simulink model "btp_gas_networkmodel"  (R2020a)
settings: Solver=VariableStepAuto  StartTime=0.0  StopTime=1e5  RelTol=1e-3
PreLoadFcn:
  | building_length = 15; % m
  | building_width = 10; % m
  | building_height = 2.5; % m
  | 
  | wall_thickness = 0.2; % m
  | wall_density = 2000; % kg/m^3
  | wall_specific_heat = 840; % J/(kg*K)
  | wall_conductivity = 0.04; % W/(m*K)
  | wall_heat_transfer_coeff_internal = 25; % W/(m^2*K)
  | wall_heat_transfer_coeff_external = 35; % W/(m^2*K)
  | 
  | roof_thickness = 0.2; % m
  | roof_density = 2000; % kg/m^3
  | roof_specific_heat = 840; % J/(kg*K)
  | roof_conductivity = 0.035; % W/(m*K)
  | roof_heat_transfer_coeff_internal = 10; % W/(m^2*K)
  | roof_heat_transfer_coeff_external = 30; % W/(m^2*K)
  | 
  | floor_thickness = 0.1; % m
  | floor_conductivity = 0.15; % W/(m*K)
  | floor_heat_transfer_coeff_internal = 15; % W/(m^2*K)
  | 
  | door_area = 2*0.6; % m^2
  | 
  | duct_area = 0.1^2; % m^2
  | 
  | fan_setting_table = 0 : 4; % 1
  | fan_flow_rate_table = [0 0.08 0.12 0.16 0.2]; % kg/s
  | 
  | initial_temperature = 35; % degC
  | ground_temperature = 25; % degC
  | 
  | flow_reversal_Mach = 1e-5; % 1
InitFcn:
  | zone_volume = building_length * building_width * building_height / 4; % m^3
  | zone_flow_area = 0.7 * building_height * (building_length + building_width) / 4; % m^2
undefined symbols (not defined in the file): sigbuilder_block
libraries: fl_lib x49, nesl_utility x15
(part 2 of 2)

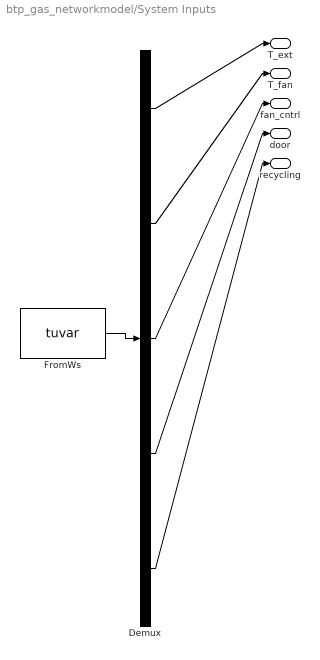
== system btp_gas_networkmodel/System Inputs ==
  Demux : Demux  Tag=STV Demux  Outputs=5
      settings: DisplayOption=none
  FromWs : FromWorkspace  Tag=STV FromWs  VariableName=tuvar
      SigBuilderData=|
      | common.afterFinalStr = 'Extrapolate'
      | common.sampleTime = 0
      | dataSet(1).timeRange = [0 100000]
      | dataSet(1).name = 'Fan Control'
      | dataSet(2).timeRange = [0 100000]
      | dataSet(2).name = 'Fan Temperature'
      | dataSet(3).timeRange = [0 100000]
      | dataSet(3).name = 'Disturbances'
      | sbobj.Groups(1).Name = 'Fan Control'
      | sbobj.Groups(1).Signals(1).Name = 'T_ext'
      | sbobj.Groups(1).Signals(1).XData = [0 100000]
      | sbobj.Groups(1).Signals(1).YData = [35 35]
      | sbobj.Groups(1).Signals(2).Name = 'T_fan'
      | sbobj.Groups(1).Signals(2).XData = [0 100000]
      | sbobj.Groups(1).Signals(2).YData = [20 20]
      | sbobj.Groups(1).Signals(3).Name = 'fan_cntrl'
      | sbobj.Groups(1).Signals(3).XData = [0 20000 20000 40000 40000 60000 80000 100000]
      | sbobj.Groups(1).Signals(3).YData = [1 1 2 2 1 1 1 1]
      | sbobj.Groups(1).Signals(4).Name = 'door'
      | sbobj.Groups(1).Signals(4).XData = [0 100000]
      | sbobj.Groups(1).Signals(4).YData = [0 0]
      | sbobj.Groups(1).Signals(5).Name = 'recycling'
      | sbobj.Groups(1).Signals(5).XData = [0 100000]
      | sbobj.Groups(1).Signals(5).YData = [0 0]
      | sbobj.Groups(1).TimeRange = [0 100000]
      | sbobj.Groups(2).Name = 'Fan Temperature'
      | sbobj.Groups(2).Signals(1).Name = 'T_ext'
      | sbobj.Groups(2).Signals(1).XData = [0 100000]
      | sbobj.Groups(2).Signals(1).YData = [35 35]
      | sbobj.Groups(2).Signals(2).Name = 'T_fan'
      | sbobj.Groups(2).Signals(2).XData = [0 20000 20000 40000 40000 60000 60000 80000 80000 100000]
      | sbobj.Groups(2).Signals(2).YData = [20 20 15 15 20 20 35 35 20 20]
      | sbobj.Groups(2).Signals(3).Name = 'fan_cntrl'
      | sbobj.Groups(2).Signals(3).XData = [0 100000]
      | sbobj.Groups(2).Signals(3).YData = [1 1]
      | sbobj.Groups(2).Signals(4).Name = 'door'
      | sbobj.Groups(2).Signals(4).XData = [0 100000]
      | sbobj.Groups(2).Signals(4).YData = [0 0]
      | sbobj.Groups(2).Signals(5).Name = 'recycling'
      | sbobj.Groups(2).Signals(5).XData = [0 100000]
      | sbobj.Groups(2).Signals(5).YData = [0 0]
      | sbobj.Groups(2).TimeRange = [0 100000]
      | sbobj.Groups(3).Name = 'Disturbances'
      | sbobj.Groups(3).Signals(1).Name = 'T_ext'
      | sbobj.Groups(3).Signals(1).XData = [0 100000]
      | sbobj.Groups(3).Signals(1).YData = [35 35]
      | sbobj.Groups(3).Signals(2).Name = 'T_fan'
      | sbobj.Groups(3).Signals(2).XData = [0 100000]
      | sbobj.Groups(3).Signals(2).YData = [20 20]
      | sbobj.Groups(3).Signals(3).Name = 'fan_cntrl'
      | sbobj.Groups(3).Signals(3).XData = [0 100000]
      | sbobj.Groups(3).Signals(3).YData = [1 1]
      | sbobj.Groups(3).Signals(4).Name = 'door'
      | sbobj.Groups(3).Signals(4).XData = [0 20000 30000 40000 100000]
      | sbobj.Groups(3).Signals(4).YData = [0 0 1 0 0]
      | sbobj.Groups(3).Signals(5).Name = 'recycling'
      | sbobj.Groups(3).Signals(5).XData = [0 60000 60000 80000 80000 100000]
      | sbobj.Groups(3).Signals(5).YData = [0 0 0.5 0.5 0 0]
      | sbobj.Groups(3).TimeRange = [0 100000]
  T_ext : Outport  Tag=STV Outport  VectorParamsAs1DForOutWhenUnconnected=off
  T_fan : Outport  Tag=STV Outport  Port=2  VectorParamsAs1DForOutWhenUnconnected=off
  fan_cntrl : Outport  Tag=STV Outport  Port=3  VectorParamsAs1DForOutWhenUnconnected=off
  door : Outport  Tag=STV Outport  Port=4  VectorParamsAs1DForOutWhenUnconnected=off
  recycling : Outport  Tag=STV Outport  Port=5  VectorParamsAs1DForOutWhenUnconnected=off
  wires:
  FromWs/1 -> Demux/1
  Demux/1 -> T_ext/1
  Demux/2 -> T_fan/1
  Demux/3 -> fan_cntrl/1
  Demux/4 -> door/1
  Demux/5 -> recycling/1

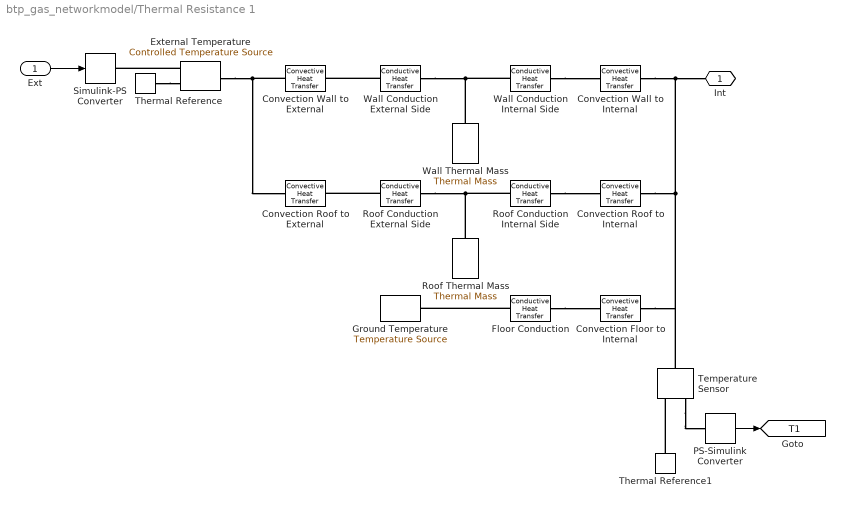
== system btp_gas_networkmodel/Thermal Resistance 1 ==
  Ext : Inport
  Convection Floor to Internal : fl_lib/Thermal/Thermal Elements/Convective Heat Transfer  area=floor_area m^2  heat_tr_coeff=floor_heat_transfer_coeff_internal W/(m^2 * K)  T_specify=off  T_priority=None  T=0 K  T_nominal_specify=off  T_nominal_unit=K  T_nominal_value=1  Q_specify=off  Q_priority=None  Q=0 W  Q_nominal_specify=off  Q_nominal_unit=W  Q_nominal_value=1
  Convection Roof to External : fl_lib/Thermal/Thermal Elements/Convective Heat Transfer  area=roof_area m^2  heat_tr_coeff=roof_heat_transfer_coeff_external W/(m^2 * K)  T_specify=off  T_priority=None  T=0 K  T_nominal_specify=off  T_nominal_unit=K  T_nominal_value=1  Q_specify=off  Q_priority=None  Q=0 W  Q_nominal_specify=off  Q_nominal_unit=W  Q_nominal_value=1
  Convection Roof to Internal : fl_lib/Thermal/Thermal Elements/Convective Heat Transfer  area=roof_area m^2  heat_tr_coeff=roof_heat_transfer_coeff_internal W/(m^2 * K)  T_specify=off  T_priority=None  T=0 K  T_nominal_specify=off  T_nominal_unit=K  T_nominal_value=1  Q_specify=off  Q_priority=None  Q=0 W  Q_nominal_specify=off  Q_nominal_unit=W  Q_nominal_value=1
  Convection Wall to External : fl_lib/Thermal/Thermal Elements/Convective Heat Transfer  area=wall_area m^2  heat_tr_coeff=wall_heat_transfer_coeff_external W/(m^2 * K)  T_specify=off  T_priority=None  T=0 K  T_nominal_specify=off  T_nominal_unit=K  T_nominal_value=1  Q_specify=off  Q_priority=None  Q=0 W  Q_nominal_specify=off  Q_nominal_unit=W  Q_nominal_value=1
  Convection Wall to Internal : fl_lib/Thermal/Thermal Elements/Convective Heat Transfer  area=wall_area m^2  heat_tr_coeff=wall_heat_transfer_coeff_internal W/(m^2 * K)  T_specify=off  T_priority=None  T=0 K  T_nominal_specify=off  T_nominal_unit=K  T_nominal_value=1  Q_specify=off  Q_priority=None  Q=0 W  Q_nominal_specify=off  Q_nominal_unit=W  Q_nominal_value=1
  External Temperature : fl_lib/Thermal/Thermal Sources/Controlled Temperature Source
  Floor Conduction : fl_lib/Thermal/Thermal Elements/Conductive Heat Transfer  area=floor_area m^2  thickness=floor_thickness m  th_cond=floor_conductivity W/(m*K)  T_specify=off  T_priority=None  T=0 K  T_nominal_specify=off  T_nominal_unit=K  T_nominal_value=1  Q_specify=off  Q_priority=None  Q=0 W  Q_nominal_specify=off  Q_nominal_unit=W  Q_nominal_value=1
  Ground Temperature : fl_lib/Thermal/Thermal Sources/Temperature Source  temperature=ground_temperature degC
  PS-Simulink Converter : nesl_utility/PS-Simulink Converter  PhysicalDomain=network_engine_domain  SubClassName=ps_output  LeftPortType=input  RightPortType=output  PseudoPeriodic=off  Frequencies=[]  Unit=degC  AffineConversion=on
  Roof Conduction External Side : fl_lib/Thermal/Thermal Elements/Conductive Heat Transfer  area=roof_area m^2  thickness=roof_thickness / 2 m  th_cond=roof_conductivity W/(m*K)  T_specify=off  T_priority=None  T=0 K  T_nominal_specify=off  T_nominal_unit=K  T_nominal_value=1  Q_specify=off  Q_priority=None  Q=0 W  Q_nominal_specify=off  Q_nominal_unit=W  Q_nominal_value=1
  Roof Conduction Internal Side : fl_lib/Thermal/Thermal Elements/Conductive Heat Transfer  area=roof_area m^2  thickness=roof_thickness / 2 m  th_cond=roof_conductivity W/(m*K)  T_specify=off  T_priority=None  T=0 K  T_nominal_specify=off  T_nominal_unit=K  T_nominal_value=1  Q_specify=off  Q_priority=None  Q=0 W  Q_nominal_specify=off  Q_nominal_unit=W  Q_nominal_value=1
  Roof Thermal Mass : fl_lib/Thermal/Thermal Elements/Thermal Mass  mass=roof_area * roof_thickness * wall_density kg  sp_heat=roof_specific_heat J/kg/K  T_specify=on  T_priority=High  T=roof_initial_temperature degC  T_nominal_specify=off  T_nominal_unit=K  T_nominal_value=1  Q_specify=off  Q_priority=None  Q=0 W  Q_nominal_specify=off  Q_nominal_unit=W  Q_nominal_value=1
  Simulink-PS Converter : nesl_utility/Simulink-PS Converter  PhysicalDomain=network_engine_domain  SubClassName=ps_input  LeftPortType=input  RightPortType=output  PseudoPeriodic=off  Frequencies=[]  NoiseDistribution=none  NoiseParameters=[]  Unit=degC  AffineConversion=on  FilteringAndDerivatives=provide  SimscapeFilterOrder=1  InputFilterTimeConstant=0.001  UdotUserProvided=0
  Temperature Sensor : fl_lib/Thermal/Thermal Sensors/Temperature Sensor
  Thermal Reference : fl_lib/Thermal/Thermal Elements/Thermal Reference
  Thermal Reference1 : fl_lib/Thermal/Thermal Elements/Thermal Reference
  Wall Conduction External Side : fl_lib/Thermal/Thermal Elements/Conductive Heat Transfer  area=wall_area m^2  thickness=wall_thickness / 2 m  th_cond=wall_conductivity W/(m*K)  T_specify=off  T_priority=None  T=0 K  T_nominal_specify=off  T_nominal_unit=K  T_nominal_value=1  Q_specify=off  Q_priority=None  Q=0 W  Q_nominal_specify=off  Q_nominal_unit=W  Q_nominal_value=1
  Wall Conduction Internal Side : fl_lib/Thermal/Thermal Elements/Conductive Heat Transfer  area=wall_area m^2  thickness=wall_thickness / 2 m  th_cond=wall_conductivity W/(m*K)  T_specify=off  T_priority=None  T=0 K  T_nominal_specify=off  T_nominal_unit=K  T_nominal_value=1  Q_specify=off  Q_priority=None  Q=0 W  Q_nominal_specify=off  Q_nominal_unit=W  Q_nominal_value=1
  Wall Thermal Mass : fl_lib/Thermal/Thermal Elements/Thermal Mass  mass=wall_area * wall_thickness * wall_density kg  sp_heat=wall_specific_heat J/kg/K  T_specify=on  T_priority=High  T=wall_initial_temperature degC  T_nominal_specify=off  T_nominal_unit=K  T_nominal_value=1  Q_specify=off  Q_priority=None  Q=0 W  Q_nominal_specify=off  Q_nominal_unit=W  Q_nominal_value=1
  Int : PMIOPort  Side=Right
  tag scope: T1=global
  wires:
  Ext/1 -> Simulink-PS Converter/1
  PS-Simulink Converter/1 -> [T1]
  connections:
  External Temperature/RConn1 -- Simulink-PS Converter/RConn1
  Wall Conduction Internal Side/RConn1 -- Convection Wall to Internal/LConn1
  Convection Roof to Internal/RConn1 -- Convection Floor to Internal/RConn1 -- Temperature Sensor/LConn1 -- Convection Wall to Internal/RConn1 -- Int/RConn1
  External Temperature/LConn1 -- Convection Wall to External/LConn1 -- Convection Roof to External/LConn1
  Wall Conduction External Side/LConn1 -- Convection Wall to External/RConn1
  Wall Thermal Mass/LConn1 -- Wall Conduction Internal Side/LConn1 -- Wall Conduction External Side/RConn1
  Roof Thermal Mass/LConn1 -- Roof Conduction Internal Side/LConn1 -- Roof Conduction External Side/RConn1
  Roof Conduction External Side/LConn1 -- Convection Roof to External/RConn1
  Roof Conduction Internal Side/RConn1 -- Convection Roof to Internal/LConn1
  Floor Conduction/RConn1 -- Convection Floor to Internal/LConn1
  Floor Conduction/LConn1 -- Ground Temperature/LConn1
  Thermal Reference1/LConn1 -- Temperature Sensor/RConn1
  Temperature Sensor/RConn2 -- PS-Simulink Converter/LConn1
  Thermal Reference/LConn1 -- External Temperature/RConn2

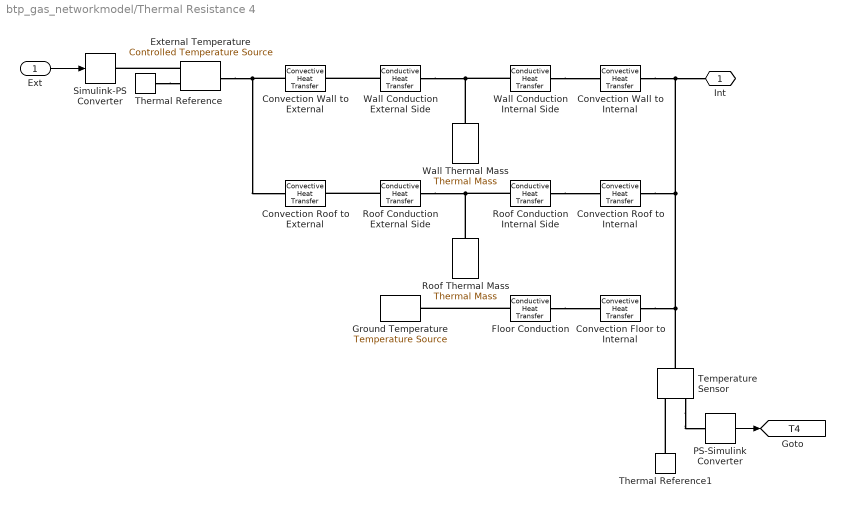
== system btp_gas_networkmodel/Thermal Resistance 4 ==
  Ext : Inport
  Convection Floor to Internal : fl_lib/Thermal/Thermal Elements/Convective Heat Transfer  area=floor_area m^2  heat_tr_coeff=floor_heat_transfer_coeff_internal W/(m^2 * K)  T_specify=off  T_priority=None  T=0 K  T_nominal_specify=off  T_nominal_unit=K  T_nominal_value=1  Q_specify=off  Q_priority=None  Q=0 W  Q_nominal_specify=off  Q_nominal_unit=W  Q_nominal_value=1
  Convection Roof to External : fl_lib/Thermal/Thermal Elements/Convective Heat Transfer  area=roof_area m^2  heat_tr_coeff=roof_heat_transfer_coeff_external W/(m^2 * K)  T_specify=off  T_priority=None  T=0 K  T_nominal_specify=off  T_nominal_unit=K  T_nominal_value=1  Q_specify=off  Q_priority=None  Q=0 W  Q_nominal_specify=off  Q_nominal_unit=W  Q_nominal_value=1
  Convection Roof to Internal : fl_lib/Thermal/Thermal Elements/Convective Heat Transfer  area=roof_area m^2  heat_tr_coeff=roof_heat_transfer_coeff_internal W/(m^2 * K)  T_specify=off  T_priority=None  T=0 K  T_nominal_specify=off  T_nominal_unit=K  T_nominal_value=1  Q_specify=off  Q_priority=None  Q=0 W  Q_nominal_specify=off  Q_nominal_unit=W  Q_nominal_value=1
  Convection Wall to External : fl_lib/Thermal/Thermal Elements/Convective Heat Transfer  area=wall_area m^2  heat_tr_coeff=wall_heat_transfer_coeff_external W/(m^2 * K)  T_specify=off  T_priority=None  T=0 K  T_nominal_specify=off  T_nominal_unit=K  T_nominal_value=1  Q_specify=off  Q_priority=None  Q=0 W  Q_nominal_specify=off  Q_nominal_unit=W  Q_nominal_value=1
  Convection Wall to Internal : fl_lib/Thermal/Thermal Elements/Convective Heat Transfer  area=wall_area m^2  heat_tr_coeff=wall_heat_transfer_coeff_internal W/(m^2 * K)  T_specify=off  T_priority=None  T=0 K  T_nominal_specify=off  T_nominal_unit=K  T_nominal_value=1  Q_specify=off  Q_priority=None  Q=0 W  Q_nominal_specify=off  Q_nominal_unit=W  Q_nominal_value=1
  External Temperature : fl_lib/Thermal/Thermal Sources/Controlled Temperature Source
  Floor Conduction : fl_lib/Thermal/Thermal Elements/Conductive Heat Transfer  area=floor_area m^2  thickness=floor_thickness m  th_cond=floor_conductivity W/(m*K)  T_specify=off  T_priority=None  T=0 K  T_nominal_specify=off  T_nominal_unit=K  T_nominal_value=1  Q_specify=off  Q_priority=None  Q=0 W  Q_nominal_specify=off  Q_nominal_unit=W  Q_nominal_value=1
  Ground Temperature : fl_lib/Thermal/Thermal Sources/Temperature Source  temperature=ground_temperature degC
  PS-Simulink Converter : nesl_utility/PS-Simulink Converter  PhysicalDomain=network_engine_domain  SubClassName=ps_output  LeftPortType=input  RightPortType=output  PseudoPeriodic=off  Frequencies=[]  Unit=degC  AffineConversion=on
  Roof Conduction External Side : fl_lib/Thermal/Thermal Elements/Conductive Heat Transfer  area=roof_area m^2  thickness=roof_thickness / 2 m  th_cond=roof_conductivity W/(m*K)  T_specify=off  T_priority=None  T=0 K  T_nominal_specify=off  T_nominal_unit=K  T_nominal_value=1  Q_specify=off  Q_priority=None  Q=0 W  Q_nominal_specify=off  Q_nominal_unit=W  Q_nominal_value=1
  Roof Conduction Internal Side : fl_lib/Thermal/Thermal Elements/Conductive Heat Transfer  area=roof_area m^2  thickness=roof_thickness / 2 m  th_cond=roof_conductivity W/(m*K)  T_specify=off  T_priority=None  T=0 K  T_nominal_specify=off  T_nominal_unit=K  T_nominal_value=1  Q_specify=off  Q_priority=None  Q=0 W  Q_nominal_specify=off  Q_nominal_unit=W  Q_nominal_value=1
  Roof Thermal Mass : fl_lib/Thermal/Thermal Elements/Thermal Mass  mass=roof_area * roof_thickness * wall_density kg  sp_heat=roof_specific_heat J/kg/K  T_specify=on  T_priority=High  T=roof_initial_temperature degC  T_nominal_specify=off  T_nominal_unit=K  T_nominal_value=1  Q_specify=off  Q_priority=None  Q=0 W  Q_nominal_specify=off  Q_nominal_unit=W  Q_nominal_value=1
  Simulink-PS Converter : nesl_utility/Simulink-PS Converter  PhysicalDomain=network_engine_domain  SubClassName=ps_input  LeftPortType=input  RightPortType=output  PseudoPeriodic=off  Frequencies=[]  NoiseDistribution=none  NoiseParameters=[]  Unit=degC  AffineConversion=on  FilteringAndDerivatives=provide  SimscapeFilterOrder=1  InputFilterTimeConstant=0.001  UdotUserProvided=0
  Temperature Sensor : fl_lib/Thermal/Thermal Sensors/Temperature Sensor
  Thermal Reference : fl_lib/Thermal/Thermal Elements/Thermal Reference
  Thermal Reference1 : fl_lib/Thermal/Thermal Elements/Thermal Reference
  Wall Conduction External Side : fl_lib/Thermal/Thermal Elements/Conductive Heat Transfer  area=wall_area m^2  thickness=wall_thickness / 2 m  th_cond=wall_conductivity W/(m*K)  T_specify=off  T_priority=None  T=0 K  T_nominal_specify=off  T_nominal_unit=K  T_nominal_value=1  Q_specify=off  Q_priority=None  Q=0 W  Q_nominal_specify=off  Q_nominal_unit=W  Q_nominal_value=1
  Wall Conduction Internal Side : fl_lib/Thermal/Thermal Elements/Conductive Heat Transfer  area=wall_area m^2  thickness=wall_thickness / 2 m  th_cond=wall_conductivity W/(m*K)  T_specify=off  T_priority=None  T=0 K  T_nominal_specify=off  T_nominal_unit=K  T_nominal_value=1  Q_specify=off  Q_priority=None  Q=0 W  Q_nominal_specify=off  Q_nominal_unit=W  Q_nominal_value=1
  Wall Thermal Mass : fl_lib/Thermal/Thermal Elements/Thermal Mass  mass=wall_area * wall_thickness * wall_density kg  sp_heat=wall_specific_heat J/kg/K  T_specify=on  T_priority=High  T=wall_initial_temperature degC  T_nominal_specify=off  T_nominal_unit=K  T_nominal_value=1  Q_specify=off  Q_priority=None  Q=0 W  Q_nominal_specify=off  Q_nominal_unit=W  Q_nominal_value=1
  Int : PMIOPort  Side=Right
  tag scope: T4=global
  wires:
  PS-Simulink Converter/1 -> [T4]
  Ext/1 -> Simulink-PS Converter/1
  connections:
  Thermal Reference/LConn1 -- External Temperature/RConn2
  Temperature Sensor/RConn2 -- PS-Simulink Converter/LConn1
  Thermal Reference1/LConn1 -- Temperature Sensor/RConn1
  Floor Conduction/LConn1 -- Ground Temperature/LConn1
  Floor Conduction/RConn1 -- Convection Floor to Internal/LConn1
  Roof Conduction Internal Side/RConn1 -- Convection Roof to Internal/LConn1
  Roof Conduction External Side/LConn1 -- Convection Roof to External/RConn1
  Roof Conduction Internal Side/LConn1 -- Roof Thermal Mass/LConn1 -- Roof Conduction External Side/RConn1
  Wall Conduction Internal Side/LConn1 -- Wall Thermal Mass/LConn1 -- Wall Conduction External Side/RConn1
  Wall Conduction External Side/LConn1 -- Convection Wall to External/RConn1
  Convection Wall to External/LConn1 -- Convection Roof to External/LConn1 -- External Temperature/LConn1
  Convection Floor to Internal/RConn1 -- Int/RConn1 -- Convection Wall to Internal/RConn1 -- Convection Roof to Internal/RConn1 -- Temperature Sensor/LConn1
  Wall Conduction Internal Side/RConn1 -- Convection Wall to Internal/LConn1
  External Temperature/RConn1 -- Simulink-PS Converter/RConn1

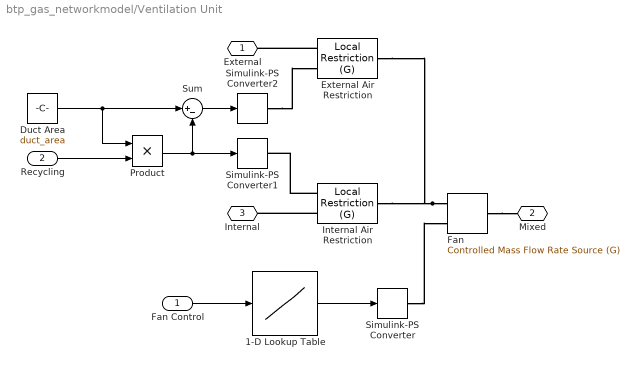
== system btp_gas_networkmodel/Ventilation Unit ==
  Fan Control : Inport
  Recycling : Inport  Port=2
  1-D Lookup Table : Lookup_n-D  NumberOfTableDimensions=1  BreakpointsForDimension1=fan_setting_table  Table=fan_flow_rate_table  ExtrapMethod=Clip  InternalRulePriority=Speed  RndMeth=Simplest  InputSameDT=on
  Duct Area : Constant  Value=duct_area
  External Air Restriction : fl_lib/Gas/Elements/Local Restriction (G)  restriction_type=foundation.enum.restriction_type.variable  restriction_area=1e-3 m^2  min_area=1e-10 m^2  max_area=0.99 * duct_area m^2  area=duct_area m^2  Cd=0.8  B_lam=0.999
      settings: SourceProductBaseCode=SS  InternalSimscapePortConfiguration="{\"Bottom\":[],\"Left\":[{\"id\":\"A\",\"label\":\"A\",\"type\":\"foundation.gas.gas\"},{\"id\":\"area_in\",\"label\":\"AR\",\"type\":\"input\"}],\"Right\":[{\"id\":\"B\",\"label\":\"B\",\"type\":\"foundation.gas.gas\"}],\"Top\":[]}"
  Fan : fl_lib/Gas/Sources/Controlled Mass Flow Rate Source (G)  power_spec=1  area_A=duct_area m^2  area_B=duct_area m^2
      settings: SourceProductName=Foundation Library  InternalSimscapePortConfiguration="{\"Bottom\":[],\"Left\":[{\"id\":\"A\",\"label\":\"A\",\"type\":\"foundation.gas.gas\"},{\"id\":\"M\",\"label\":\"M\",\"type\":\"input\"}],\"Right\":[{\"id\":\"B\",\"label\":\"B\",\"type\":\"foundation.gas.gas\"}],\"Top\":[]}"
  Internal Air Restriction : fl_lib/Gas/Elements/Local Restriction (G)  restriction_type=foundation.enum.restriction_type.variable  restriction_area=1e-3 m^2  min_area=1e-10 m^2  max_area=0.99 * duct_area m^2  area=duct_area m^2  Cd=0.8  B_lam=0.999
      settings: SourceProductBaseCode=SS  InternalSimscapePortConfiguration="{\"Bottom\":[],\"Left\":[{\"id\":\"A\",\"label\":\"A\",\"type\":\"foundation.gas.gas\"},{\"id\":\"area_in\",\"label\":\"AR\",\"type\":\"input\"}],\"Right\":[{\"id\":\"B\",\"label\":\"B\",\"type\":\"foundation.gas.gas\"}],\"Top\":[]}"
  Product : Product
  Simulink-PS Converter : nesl_utility/Simulink-PS Converter  PhysicalDomain=network_engine_domain  SubClassName=ps_input  LeftPortType=input  RightPortType=output  PseudoPeriodic=off  Frequencies=[]  NoiseDistribution=none  NoiseParameters=[]  Unit=kg/s  AffineConversion=off  FilteringAndDerivatives=provide  SimscapeFilterOrder=1  InputFilterTimeConstant=0.001  UdotUserProvided=0
  Simulink-PS Converter1 : nesl_utility/Simulink-PS Converter  PhysicalDomain=network_engine_domain  SubClassName=ps_input  LeftPortType=input  RightPortType=output  PseudoPeriodic=off  Frequencies=[]  NoiseDistribution=none  NoiseParameters=[]  Unit=m^2  AffineConversion=off  FilteringAndDerivatives=provide  SimscapeFilterOrder=1  InputFilterTimeConstant=0.001  UdotUserProvided=0
  Simulink-PS Converter2 : nesl_utility/Simulink-PS Converter  PhysicalDomain=network_engine_domain  SubClassName=ps_input  LeftPortType=input  RightPortType=output  PseudoPeriodic=off  Frequencies=[]  NoiseDistribution=none  NoiseParameters=[]  Unit=m^2  AffineConversion=off  FilteringAndDerivatives=provide  SimscapeFilterOrder=1  InputFilterTimeConstant=0.001  UdotUserProvided=0
  Sum : Sum  Inputs=|+-
  External : PMIOPort  Side=Left
  Mixed : PMIOPort  Port=2  Side=Right
  Internal : PMIOPort  Port=3  Side=Left
  wires:
  Fan Control/1 -> 1-D Lookup Table/1
  1-D Lookup Table/1 -> Simulink-PS Converter/1
  Recycling/1 -> Product/2
  Product/1 -> Sum/2, Simulink-PS Converter1/1
  Sum/1 -> Simulink-PS Converter2/1
  Duct Area/1 -> Sum/1, Product/1
  connections:
  Fan/RConn1 -- Mixed/RConn1
  Simulink-PS Converter/RConn1 -- Fan/LConn2
  Fan/LConn1 -- Internal Air Restriction/RConn1 -- External Air Restriction/RConn1
  Internal Air Restriction/LConn2 -- Simulink-PS Converter1/RConn1
  Simulink-PS Converter2/RConn1 -- External Air Restriction/LConn2
  Internal Air Restriction/LConn1 -- Internal/RConn1
  External Air Restriction/LConn1 -- External/RConn1
